simulink model "observer_down_model"  (R2024a)
settings: Solver=FixedStepAuto  StartTime=0.0  StopTime=2  FixedStep=0.0001  RelTol=1e-3
values from neighbouring files (symbols this model uses):
  A = [5 -5 -9 3; -5 5 -3 9; -9 -3 5 5; 3 9 5 5]    [ex.m]    (also in observer.m = [20 5 -16 9; 6 1 -4 1; 32 9 -25 14; 8 4 -6 4]; observer_down.m; reg.m = [2 3; -3 2])
  B = [2; 6; 6; 2]    [ex.m]    (also in observer_down.m; reg.m = [0; -4])
  C = [1 -1 1 1; 1 3 -1 3]    [ex.m]    (also in observer.m = [-1 0 1 -1]; observer_down.m = [0 0 0 1; 0 1 0 0])
  CQ = [C; Q]    [observer_down.m]
  D = [2; 1]    [ex.m]    (also in observer_down.m)
  G = [-5 0; 0 -6]    [observer_down.m]
  K = -Yr*Pr^(-1)    [ex.m]    (also in observer_down.m)
  Q = sylvester(G, -A, Y*C)    [observer_down.m]
  Y = [-5 0; 1 0]    [observer_down.m]
settings Model: Creator=ventus  LastModifiedBy=ventus

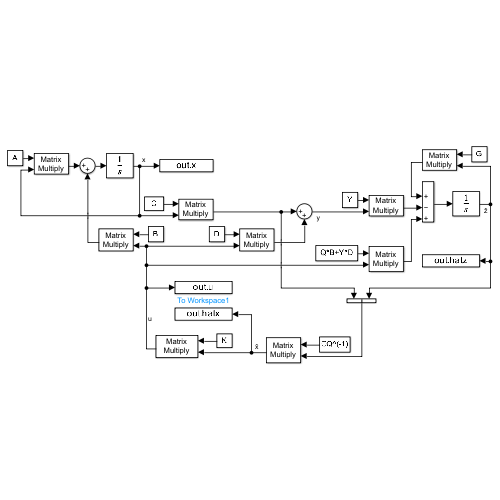
[thumbnail: Simulink's stored preview of the top-level diagram]
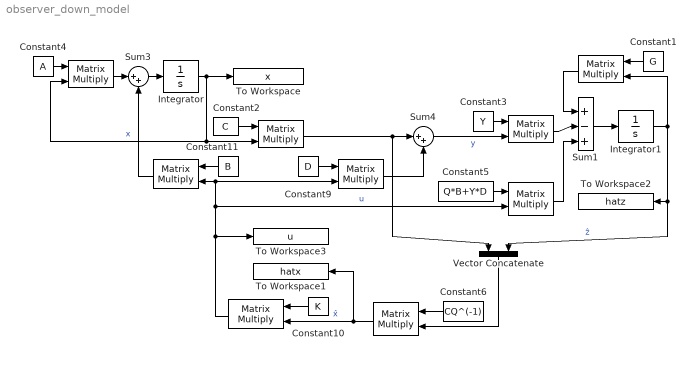
== system observer_down_model ==
  "   " : Product  Multiplication=Matrix(*)
  "     " : Product  Multiplication=Matrix(*)
  "        " : Product  Multiplication=Matrix(*)
  "                " : Product  Multiplication=Matrix(*)
  "                  " : Product  Multiplication=Matrix(*)
  "                   " : Product  Multiplication=Matrix(*)
  "                    " : Product  Multiplication=Matrix(*)
  "                     " : Product  Multiplication=Matrix(*)
  "                      " : Product  Multiplication=Matrix(*)
  Constant1 : Constant  Value=G  VectorParams1D=off
  Constant10 : Constant  Value=K  VectorParams1D=off
  Constant11 : Constant  Value=B  VectorParams1D=off
  Constant2 : Constant  Value=C  VectorParams1D=off
  Constant3 : Constant  Value=Y  VectorParams1D=off
  Constant4 : Constant  Value=A  VectorParams1D=off
  Constant5 : Constant  Value=Q*B+Y*D  VectorParams1D=off
  Constant6 : Constant  Value=CQ^(-1)  VectorParams1D=off
  Constant9 : Constant  Value=D  VectorParams1D=off
  Integrator : Integrator  InitialCondition=[1; 1; 1; 1]
  Integrator1 : Integrator  InitialCondition=[0; 0]
  Sum1 : Sum  Inputs=|+-+
  Sum3 : Sum  Inputs=|++
  Sum4 : Sum  Inputs=|++
  To Workspace : ToWorkspace  VariableName=x  SaveFormat=Timeseries  SampleTime=-1
  To Workspace1 : ToWorkspace  VariableName=hatx  SaveFormat=Timeseries  SampleTime=-1
  To Workspace2 : ToWorkspace  VariableName=hatz  SaveFormat=Timeseries  SampleTime=-1
  To Workspace3 : ToWorkspace  VariableName=u  SaveFormat=Timeseries  SampleTime=-1
  Vector Concatenate : Concatenate
  wires:
  Constant11/1 -> "                     "/1
  Sum3/1 -> Integrator/1
  Constant10/1 -> "                      "/1
  Constant4/1 -> "     "/1
  "                     "/1 -> Sum3/2
  "        "/1 -> Sum4/2
  "                      "/1 -> To Workspace3/1, "        "/2, "                     "/2, "                   "/2  "u"
  "     "/1 -> Sum3/1
  Constant9/1 -> "        "/1
  Integrator/1 -> To Workspace/1, "     "/2, "   "/2  "x"
  Constant2/1 -> "   "/1
  Sum4/1 -> "                    "/2  "y"
  "                  "/1 -> To Workspace1/1, "                      "/2  "x̂"
  Constant1/1 -> "                "/1
  "                "/1 -> Sum1/1
  Sum1/1 -> Integrator1/1
  Integrator1/1 -> "                "/2, Vector Concatenate/2, To Workspace2/1  "ẑ"
  Constant3/1 -> "                    "/1
  "                    "/1 -> Sum1/2
  "                   "/1 -> Sum1/3
  Constant5/1 -> "                   "/1
  Vector Concatenate/1 -> "                  "/2
  Constant6/1 -> "                  "/1
  "   "/1 -> Vector Concatenate/1, Sum4/1
